simulink model "Boost_Converter"  (R2016a)
settings: Solver=VariableStepAuto  StartTime=0.0  StopTime=10.0  RelTol=1e-3
libraries: powerlib x9, powerlib_meascontrol x1
settings Model: Creator=GADDALA JAYARAJU  LastModifiedBy=GADDALA JAYARAJU

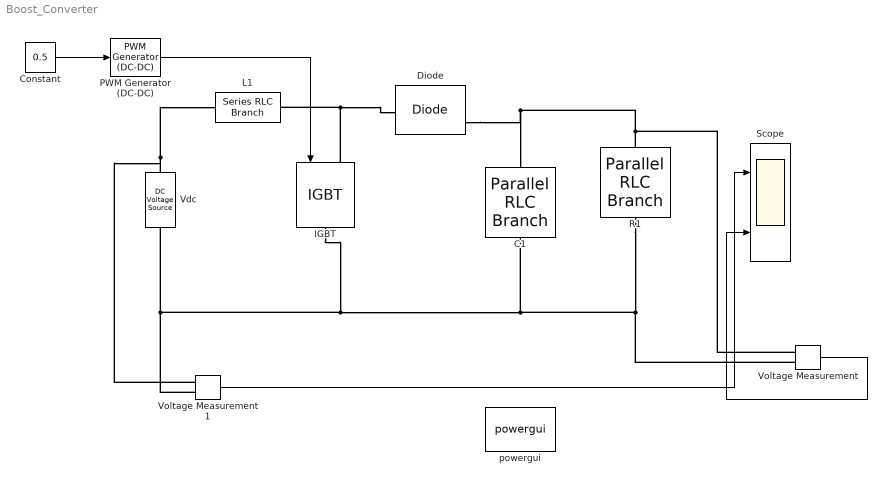
== system Boost_Converter ==
  " IGBT" : powerlib/Power Electronics/IGBT  Ron=0.01  Lon=0  Vf=1  Tf=1e-6  Tt=1e-6  IC=0  Rs=10000  Cs=inf  Measurements=off
      settings: AttributesFormatString=\n
  C1 : powerlib/Elements/Parallel RLC Branch  LConnTagsString=a  RConnTagsString=__new0  BranchType=C  Resistance=50  Inductance=1.0  SetiL0=off  InitialCurrent=0  Capacitance=33e-06  Setx0=off  InitialVoltage=0  Measurements=Branch voltage and current
  Constant : Constant  Value=0.5
  Diode : powerlib/Power Electronics/Diode  Ron=0.001  Lon=0  Vf=0.8  IC=0  UseSnubber=off  Rs=500  Cs=250e-9  Measurements=on
  L1 : powerlib/Elements/Series RLC Branch  LConnTagsString=__new0  RConnTagsString=__new0  BranchType=L  Resistance=1.0  Inductance=1e-3  SetiL0=off  InitialCurrent=0  Capacitance=1.0  Setx0=off  InitialVoltage=0  Measurements=Branch current
  PWM Generator (DC-DC) : powerlib_meascontrol/Pulse & Signal Generators/PWM Generator (DC-DC)  Fsw=31000  Ts=0
  R1 : powerlib/Elements/Parallel RLC Branch  LConnTagsString=a  RConnTagsString=__new0  BranchType=R  Resistance=50  Inductance=1.0  SetiL0=off  InitialCurrent=0  Capacitance=25e-06  Setx0=off  InitialVoltage=0  Measurements=Branch voltage and current
  Scope : Scope  NumInputPorts=2
  Vdc : powerlib/Electrical Sources/DC Voltage Source  Description=source block  Amplitude=250  Measurements=None
      settings: AttributesFormatString=\n
  Voltage Measurement : powerlib/Measurements/Voltage Measurement  PhasorSimulation=off  OutputType=Complex  PSBequivalent=0
  Voltage Measurement1 : powerlib/Measurements/Voltage Measurement  PhasorSimulation=off  OutputType=Complex  PSBequivalent=0
  powergui : powerlib/powergui  SimulationMode=Continuous  SolverType=Tustin  SampleTime=0  frequency=60  SPID=off  DisableSnubberDevices=on  DisableRonSwitches=off  DisableVfSwitches=off  SwTol=0  DisplayEquations=off  Interpol=off  ExternalGateDelay=off  methode=off  Ts=0  FunctionMessages=off  echomessages=off  HookPort=off  EnableUseOfTLC=off  x0status=blocks  frequencyindice=0  Pbase=100e6  ErrMax=1e-4  Iterations=50  UnitsV=kV  UnitsW=MW  buscounter=0  RestoreLinks=warning  ResistiveCurrentMeasurement=off  Frange=[0:2:500]  Ylog=off  Xlog=on  ShowGrid=off  save=off  variable=ZData  structure=0  ZoomFFT=on  StartTime=0.0  cycles=1  DisplayStyle=1  fundamental=60  FreqAxis=off  MaxFrequency=1000  frequencyindicesteady=1  RmsSteady=1  display=off
  wires:
  PWM Generator (DC-DC)/1 -> " IGBT"/1
  Voltage Measurement1/1 -> Scope/1
  Voltage Measurement/1 -> Scope/2
  Constant/1 -> PWM Generator (DC-DC)/1
  connections:
  " IGBT"/RConn1 -- R1/RConn1 -- Voltage Measurement/LConn2 -- C1/RConn1 -- Vdc/LConn1 -- Voltage Measurement1/LConn2
  Diode/LConn1 -- " IGBT"/LConn1 -- L1/RConn1
  Vdc/RConn1 -- L1/LConn1 -- Voltage Measurement1/LConn1
  Diode/RConn1 -- Voltage Measurement/LConn1 -- R1/LConn1 -- C1/LConn1
